simulink model "pendulum_2"  (R2024b)
settings: Solver=VariableStepAuto  StartTime=0.0  StopTime=10.0  RelTol=1e-3
values from neighbouring files (symbols this model uses):
  b = 0.1    [init_params.m]    (also in pendulum.m)
  C = 0.001    [init_params.m]    (also in pendulum.m = 0.01)
  G = 9.81    [pendulum.m]
  J = (1/3)*m*l^2    (= 0.006)    [init_params.m]    (also in pendulum.m)
  Mt = M + m    (= 0.7)    [pendulum.m]
settings Model: Creator=Ali Emir Kaplan  LastModifiedBy=Ali Emir Kaplan

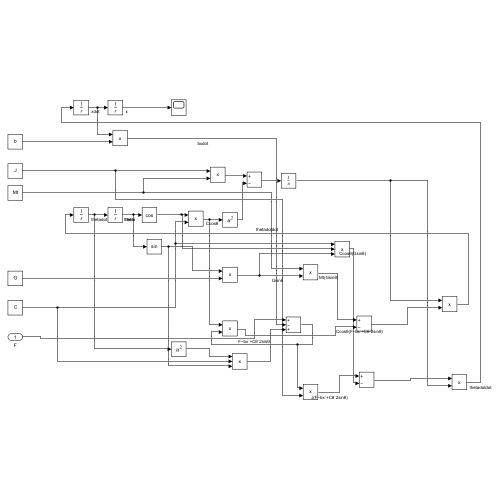
[thumbnail: Simulink's stored preview of the top-level diagram]
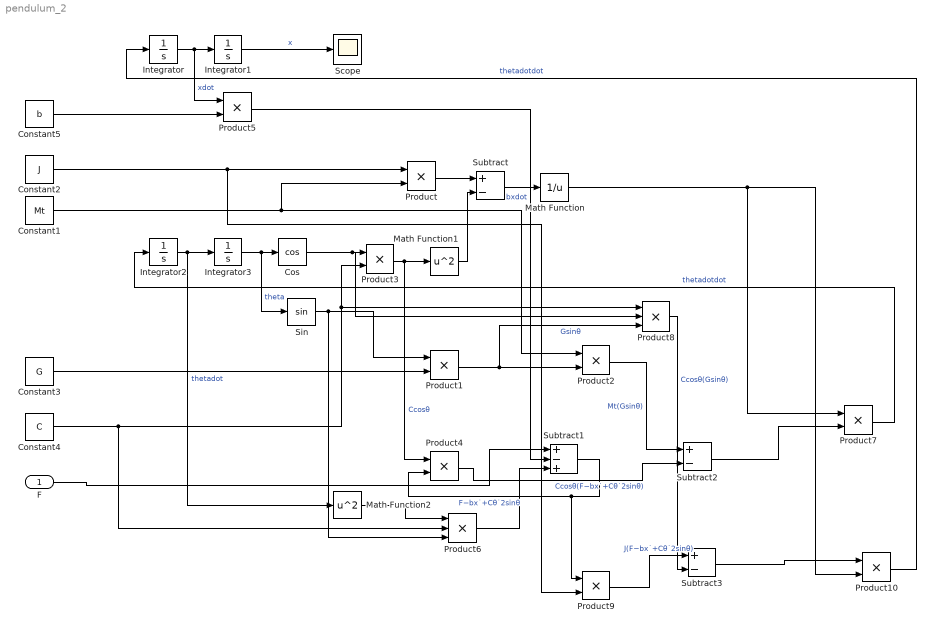
== system pendulum_2 ==
  F : Inport
  Constant1 : Constant  Value=Mt
  Constant2 : Constant  Value=J
  Constant3 : Constant  Value=G
  Constant4 : Constant  Value=C
  Constant5 : Constant  Value=b
  Cos : Trigonometry  Operator=cos
  Integrator{,1..3} (4 alike) : Integrator
  Math Function : Math  Operator=reciprocal
  Math Function1 : Math  Operator=square
  Math Function2 : Math  Operator=square
  Product{,1..5,7,9..10} (9 alike) : Product
  Product6 : Product  Inputs=3
  Product8 : Product  Inputs=3
  Scope : Scope
  Sin : Trigonometry
  Subtract : Sum  Inputs=+-
  Subtract1 : Sum  Inputs=+-+
  Subtract2 : Sum  Inputs=+-
  Subtract3 : Sum  Inputs=+-
  wires:
  Integrator3/1 -> Sin/1, Cos/1  "theta"
  Integrator2/1 -> Math Function2/1, Integrator3/1  "thetadot"
  Integrator/1 -> Product5/1, Integrator1/1  "xdot"
  Constant2/1 -> Product9/2, Product/1
  Product/1 -> Subtract/1
  Constant1/1 -> Product2/1, Product/2
  Subtract/1 -> Math Function/1
  Constant3/1 -> Product1/2
  Sin/1 -> Product6/3, Product1/1
  Product1/1 -> Product8/3, Product2/2  "Gsinθ"
  Product2/1 -> Subtract2/1  "Mt​(Gsinθ)"
  Product3/1 -> Product4/1, Math Function1/1  "Ccosθ"
  Cos/1 -> Product8/2, Product3/1
  Math Function1/1 -> Subtract/2
  Constant4/1 -> Product6/2, Product8/1, Product3/2
  Math Function/1 -> Product10/2, Product7/1
  Constant5/1 -> Product5/2
  Product5/1 -> Subtract1/2  "bxdot"
  Math Function2/1 -> Product6/1
  Product6/1 -> Subtract1/3
  F/1 -> Subtract1/1
  Subtract1/1 -> Product9/1, Product4/2  "F−bx˙+Cθ˙2sinθ"
  Product4/1 -> Subtract2/2  "Ccosθ(F−bx˙+Cθ˙2sinθ)​"
  Subtract2/1 -> Product7/2
  Product7/1 -> Integrator2/1  "thetadotdot"
  Product8/1 -> Subtract3/2  "Ccosθ(Gsinθ)"
  Product9/1 -> Subtract3/1  "J(F−bx˙+Cθ˙2sinθ)"
  Subtract3/1 -> Product10/1
  Product10/1 -> Integrator/1  "thetadotdot"
  Integrator1/1 -> Scope/1  "x"
